simulink model "test_model"  (R2020b)
settings: Solver=FixedStepAuto  StartTime=0.0  StopTime=inf  FixedStep=0.001  RelTol=1e-3
libraries: DSX_Lib x9
settings Model: PacingRate=0.450000  Creator=16047  LastModifiedBy=16047

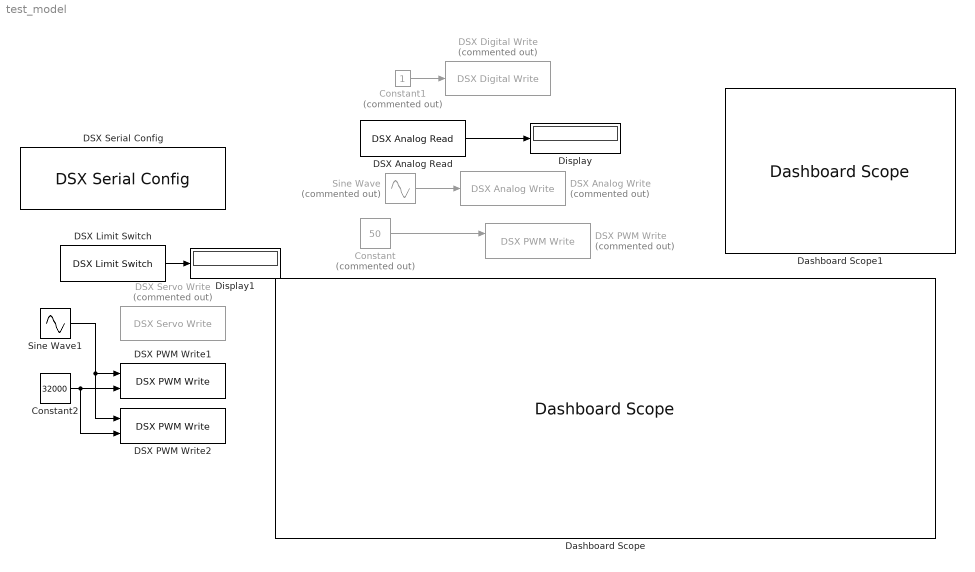
== system test_model ==
  Constant : Constant  Commented=on  Value=50
  Constant1 : Constant  Commented=on
  Constant2 : Constant  Value=32000
  DSX Analog Read : DSX_Lib/Read Blocks/DSX Analog Read  aread_pin=13
      settings: SourceProductName=DSX Library
  DSX Analog Write : DSX_Lib/Write Blocks/DSX Analog Write  Commented=on  analog_pin=17
      settings: SourceProductName=DSX Library
  DSX Digital Write : DSX_Lib/Write Blocks/DSX Digital Write  Commented=on  gpio_pin=9
      settings: SourceProductName=DSX Library
  DSX Limit Switch : DSX_Lib/Read Blocks/DSX Limit Switch  read_pin=7  emerg_stop=on
      settings: SourceProductName=DSX Library
  DSX PWM Write : DSX_Lib/Write Blocks/DSX PWM Write  Commented=on  pwm_pin=11  pwm_freq=4000
      settings: SourceProductName=DSX Library
  DSX PWM Write1 : DSX_Lib/Write Blocks/DSX PWM Write  pwm_pin=12  pwm_freq=4000
      settings: SourceProductName=DSX Library
  DSX PWM Write2 : DSX_Lib/Write Blocks/DSX PWM Write  pwm_pin=11  pwm_freq=4000
      settings: SourceProductName=DSX Library
  DSX Serial Config : DSX_Lib/DSX Serial Config  BaudRate=256000
      settings: SourceProductName=DSX Library
  DSX Servo Write : DSX_Lib/Write Blocks/DSX Servo Write  Commented=on  servo_pin=11
      settings: SourceProductName=DSX Library
  Dashboard Scope : DashboardScope  TimeSpan=10  Ymin=0  Ymax=8500
  Dashboard Scope1 : DashboardScope
  Display : Display
  Display1 : Display
  Sine Wave : Sin  Commented=on  Amplitude=1024  Bias=1024  Frequency=0.05  SampleTime=0
  Sine Wave1 : Sin  Amplitude=100  Bias=50  Frequency=0.5  SampleTime=0
  wires:
  Constant/1 -> DSX PWM Write/1
  DSX Analog Read/1 -> Display/1
  Constant1/1 -> DSX Digital Write/1
  Sine Wave/1 -> DSX Analog Write/1
  DSX Limit Switch/1 -> Display1/1
  Sine Wave1/1 -> DSX PWM Write2/1, DSX PWM Write1/1
  Constant2/1 -> DSX PWM Write2/2, DSX PWM Write1/2
